simulink model "AFASClosedloopSim"  (R2023a)
settings: Solver=FixedStepAuto  StartTime=0.0  StopTime=600  FixedStep=1/240  RelTol=1e-5
PreLoadFcn:
  | [aircraft, state] = astDehavillandBeaver();
  | thrustX = getCoefficient(aircraft,"CX","Propeller",Component="Propeller");
InitFcn:
  | AFASClosedloopSimInitialization
model workspace (MATLAB code in the model file + MAT data in the model file):
  AirReferencedVelocity = 1
  AircraftPerformance.time = 0
  AircraftPerformance.signals(1).values = [0 0 -2202]
  AircraftPerformance.signals(1).dimensions = 3
  AircraftPerformance.signals(1).label = 'CSTATE'
  AircraftPerformance.signals(1).blockName = 'asb6DOFAirframeTemplate/6DOF EOM/6DOF (Euler Angles)/xe,ye,ze'
  AircraftPerformance.signals(1).stateName = ''
  AircraftPerformance.signals(1).inReferencedModel = 0
  AircraftPerformance.signals(1).sampleTime = [0 0]
  AircraftPerformance.signals(2).values = [0.128665353089 0.259337659946 -0.178947917154]
  AircraftPerformance.signals(2).dimensions = 3
  AircraftPerformance.signals(2).label = 'CSTATE'
  AircraftPerformance.signals(2).blockName = 'asb6DOFAirframeTemplate/6DOF EOM/6DOF (Euler Angles)/Calculate DCM &
    | Euler Angles/phi
    | theta
    | psi'
  AircraftPerformance.signals(2).stateName = ''
  AircraftPerformance.signals(2).inReferencedModel = 0
  AircraftPerformance.signals(2).sampleTime = [0 0]
  AircraftPerformance.signals(3).values = [36.9119692666 8.10720863264 8.82591882596]
  AircraftPerformance.signals(3).dimensions = 3
  AircraftPerformance.signals(3).label = 'CSTATE'
  AircraftPerformance.signals(3).blockName = 'asb6DOFAirframeTemplate/6DOF EOM/6DOF (Euler Angles)/ub,vb,wb'
  AircraftPerformance.signals(3).stateName = ''
  AircraftPerformance.signals(3).inReferencedModel = 0
  AircraftPerformance.signals(3).sampleTime = [0 0]
  AircraftPerformance.signals(4).values = [0 0 0]
  AircraftPerformance.signals(4).dimensions = 3
  AircraftPerformance.signals(4).label = 'CSTATE'
  AircraftPerformance.signals(4).blockName = 'asb6DOFAirframeTemplate/6DOF EOM/6DOF (Euler Angles)/p,q,r '
  AircraftPerformance.signals(4).stateName = ''
  AircraftPerformance.signals(4).inReferencedModel = 0
  AircraftPerformance.signals(4).sampleTime = [0 0]
  AircraftPerformance.signals(5).values = [0 0]
  AircraftPerformance.signals(5).dimensions = 2
  AircraftPerformance.signals(5).label = 'CSTATE'
  AircraftPerformance.signals(5).blockName = 'asb6DOFAirframeTemplate/Environment Model/Dryden Wind Turbulence Model 
    | (Continuous (+q +r))/Filters on velocities/Hwgw(s)/wg_p1'
  AircraftPerformance.signals(5).stateName = ''
  AircraftPerformance.signals(5).inReferencedModel = 0
  AircraftPerformance.signals(5).sampleTime = [0 0]
  AircraftPerformance.signals(6).values = [0 0]
  AircraftPerformance.signals(6).dimensions = 2
  AircraftPerformance.signals(6).label = 'CSTATE'
  AircraftPerformance.signals(6).blockName = 'asb6DOFAirframeTemplate/Environment Model/Dryden Wind Turbulence Model 
    | (Continuous (+q +r))/Filters on velocities/Hwgw(s)/wg_p2'
  AircraftPerformance.signals(6).stateName = ''
  AircraftPerformance.signals(6).inReferencedModel = 0
  AircraftPerformance.signals(6).sampleTime = [0 0]
  AircraftPerformance.signals(7).values = [0 0]
  AircraftPerformance.signals(7).dimensions = 2
  AircraftPerformance.signals(7).label = 'CSTATE'
  AircraftPerformance.signals(7).blockName = 'asb6DOFAirframeTemplate/Environment Model/Dryden Wind Turbulence Model 
    | (Continuous (+q +r))/Filters on velocities/Hvgw(s)/vg_p1'
  AircraftPerformance.signals(7).stateName = ''
  AircraftPerformance.signals(7).inReferencedModel = 0
  AircraftPerformance.signals(7).sampleTime = [0 0]
  AircraftPerformance.signals(8).values = [0 0]
  AircraftPerformance.signals(8).dimensions = 2
  AircraftPerformance.signals(8).label = 'CSTATE'
  AircraftPerformance.signals(8).blockName = 'asb6DOFAirframeTemplate/Environment Model/Dryden Wind Turbulence Model 
    | (Continuous (+q +r))/Filters on velocities/Hvgw(s)/vgw_p2'
  AircraftPerformance.signals(8).stateName = ''
  AircraftPerformance.signals(8).inReferencedModel = 0
  AircraftPerformance.signals(8).sampleTime = [0 0]
  AircraftPerformance.signals(9).values = [0 0]
  AircraftPerformance.signals(9).dimensions = 2
  AircraftPerformance.signals(9).label = 'CSTATE'
  AircraftPerformance.signals(9).blockName = 'asb6DOFAirframeTemplate/Environment Model/Dryden Wind Turbulence Model 
    | (Continuous (+q +r))/Filters on velocities/Hugw(s)/ug_p'
  AircraftPerformance.signals(9).stateName = ''
  AircraftPerformance.signals(9).inReferencedModel = 0
  AircraftPerformance.signals(9).sampleTime = [0 0]
  AircraftPerformance.signals(10).values = [0 0]
  AircraftPerformance.signals(10).dimensions = 2
  AircraftPerformance.signals(10).label = 'CSTATE'
  AircraftPerformance.signals(10).blockName = 'asb6DOFAirframeTemplate/Environment Model/Dryden Wind Turbulence Model 
    | (Continuous (+q +r))/Filters on angular rates/Hrgw/rgw_p'
  AircraftPerformance.signals(10).stateName = ''
  AircraftPerformance.signals(10).inReferencedModel = 0
  AircraftPerformance.signals(10).sampleTime = [0 0]
  AircraftPerformance.signals(11).values = [0 0]
  AircraftPerformance.signals(11).dimensions = 2
  AircraftPerformance.signals(11).label = 'CSTATE'
  AircraftPerformance.signals(11).blockName = 'asb6DOFAirframeTemplate/Environment Model/Dryden Wind Turbulence Model 
    | (Continuous (+q +r))/Filters on angular rates/Hqgw/qgw_p'
  AircraftPerformance.signals(11).stateName = ''
  AircraftPerformance.signals(11).inReferencedModel = 0
  AircraftPerformance.signals(11).sampleTime = [0 0]
  AircraftPerformance.signals(12).values = [0 0]
  AircraftPerformance.signals(12).dimensions = 2
  AircraftPerformance.signals(12).label = 'CSTATE'
  AircraftPerformance.signals(12).blockName = 'asb6DOFAirframeTemplate/Environment Model/Dryden Wind Turbulence Model 
    | (Continuous (+q +r))/Filters on angular rates/Hpgw/pgw_p'
  AircraftPerformance.signals(12).stateName = ''
  AircraftPerformance.signals(12).inReferencedModel = 0
  AircraftPerformance.signals(12).sampleTime = [0 0]
  AircraftPerformance.unnamed = 0
  AircraftPerformance.type = 0
  CurrentWaypoint = 1
  FCCLatDirMode = 1
  FCCVerticalMode = 1
  FlightPlan = 1
  LookaheadDis = 15
  NextWaypoint = 1
  NumofWaypoint = 1
  OwnshipAircraftID = 1
  PreWaypoint = 1
  PreviousWaypoint = Simulink.Parameter
  PreviousWaypoint.DataType = 'auto'
  PreviousWaypoint.Complexity = 'real'
  PreviousWaypoint.Dimensions = [0 0]
  TrajectoryChange = 1
  WaypointType = 1
  inputs0.time = 0
  inputs0.signals(1).dimensions = 1
  inputs0.signals(1).values = -0.104711430294
  inputs0.signals(2).dimensions = 1
  inputs0.signals(2).values = -0.0698725229544
  inputs0.signals(3).dimensions = 1
  inputs0.signals(3).values = -0.000215042330254
  states.time = 0
  states.signals(1).values = 0
  states.signals(1).dimensions = 1
  states.signals(1).label = 'CSTATE'
  states.signals(1).blockName = 'asb6DOFAirframeTemplate/6DOF EOM/6DOF (Euler Angles)/xe,ye,ze'
  states.signals(1).stateName = 'Xe'
  states.signals(1).inReferencedModel = 0
  states.signals(1).sampleTime = [0 0]
  states.signals(2).values = 0
  states.signals(2).dimensions = 1
  states.signals(2).label = 'CSTATE'
  states.signals(2).blockName = 'asb6DOFAirframeTemplate/6DOF EOM/6DOF (Euler Angles)/xe,ye,ze'
  states.signals(2).stateName = 'Ye'
  states.signals(2).inReferencedModel = 0
  states.signals(2).sampleTime = [0 0]
  states.signals(3).values = -2202
  states.signals(3).dimensions = 1
  states.signals(3).label = 'CSTATE'
  states.signals(3).blockName = 'asb6DOFAirframeTemplate/6DOF EOM/6DOF (Euler Angles)/xe,ye,ze'
  states.signals(3).stateName = 'Ze'
  states.signals(3).inReferencedModel = 0
  states.signals(3).sampleTime = [0 0]
  states.signals(4).values = 0.128665353089
  states.signals(4).dimensions = 1
  states.signals(4).label = 'CSTATE'
  states.signals(4).blockName = 'asb6DOFAirframeTemplate/6DOF EOM/6DOF (Euler Angles)/Calculate DCM &
    | Euler Angles/phi
    | theta
    | psi'
  states.signals(4).stateName = 'phi'
  states.signals(4).inReferencedModel = 0
  states.signals(4).sampleTime = [0 0]
  states.signals(5).values = 0.259337659946
  states.signals(5).dimensions = 1
  states.signals(5).label = 'CSTATE'
  states.signals(5).blockName = 'asb6DOFAirframeTemplate/6DOF EOM/6DOF (Euler Angles)/Calculate DCM &
    | Euler Angles/phi
    | theta
    | psi'
  states.signals(5).stateName = 'theta'
  states.signals(5).inReferencedModel = 0
  states.signals(5).sampleTime = [0 0]
  states.signals(6).values = -0.178947917154
  states.signals(6).dimensions = 1
  states.signals(6).label = 'CSTATE'
  states.signals(6).blockName = 'asb6DOFAirframeTemplate/6DOF EOM/6DOF (Euler Angles)/Calculate DCM &
    | Euler Angles/phi
    | theta
    | psi'
  states.signals(6).stateName = 'psi'
  states.signals(6).inReferencedModel = 0
  states.signals(6).sampleTime = [0 0]
  states.signals(7).values = 36.9119692666
  states.signals(7).dimensions = 1
  states.signals(7).label = 'CSTATE'
  states.signals(7).blockName = 'asb6DOFAirframeTemplate/6DOF EOM/6DOF (Euler Angles)/ub,vb,wb'
  states.signals(7).stateName = 'Ubody'
  states.signals(7).inReferencedModel = 0
  states.signals(7).sampleTime = [0 0]
  states.signals(8).values = 8.10720863264
  states.signals(8).dimensions = 1
  states.signals(8).label = 'CSTATE'
  states.signals(8).blockName = 'asb6DOFAirframeTemplate/6DOF EOM/6DOF (Euler Angles)/ub,vb,wb'
  states.signals(8).stateName = 'Vbody'
  states.signals(8).inReferencedModel = 0
  states.signals(8).sampleTime = [0 0]
  states.signals(9).values = 8.82591882596
  states.signals(9).dimensions = 1
  states.signals(9).label = 'CSTATE'
  states.signals(9).blockName = 'asb6DOFAirframeTemplate/6DOF EOM/6DOF (Euler Angles)/ub,vb,wb'
  states.signals(9).stateName = 'Wbody'
  states.signals(9).inReferencedModel = 0
  states.signals(9).sampleTime = [0 0]
  states.signals(10).values = 0
  states.signals(10).dimensions = 1
  states.signals(10).label = 'CSTATE'
  states.signals(10).blockName = 'asb6DOFAirframeTemplate/6DOF EOM/6DOF (Euler Angles)/p,q,r '
  states.signals(10).stateName = 'p'
  states.signals(10).inReferencedModel = 0
  states.signals(10).sampleTime = [0 0]
  states.signals(11).values = 0
  states.signals(11).dimensions = 1
  states.signals(11).label = 'CSTATE'
  states.signals(11).blockName = 'asb6DOFAirframeTemplate/6DOF EOM/6DOF (Euler Angles)/p,q,r '
  states.signals(11).stateName = 'q'
  states.signals(11).inReferencedModel = 0
  states.signals(11).sampleTime = [0 0]
  states.signals(12).values = 0
  states.signals(12).dimensions = 1
  states.signals(12).label = 'CSTATE'
  states.signals(12).blockName = 'asb6DOFAirframeTemplate/6DOF EOM/6DOF (Euler Angles)/p,q,r '
  states.signals(12).stateName = 'r'
  states.signals(12).inReferencedModel = 0
  states.signals(12).sampleTime = [0 0]
  states.signals(13).values = [0 0]
  states.signals(13).dimensions = 2
  states.signals(13).label = 'CSTATE'
  states.signals(13).blockName = 'asb6DOFAirframeTemplate/Environment Model/Dryden Wind Turbulence Model 
    | (Continuous (+q +r))/Filters on velocities/Hwgw(s)/wg_p1'
  states.signals(13).stateName = ''
  states.signals(13).inReferencedModel = 0
  states.signals(13).sampleTime = [0 0]
  states.signals(14).values = [0 0]
  states.signals(14).dimensions = 2
  states.signals(14).label = 'CSTATE'
  states.signals(14).blockName = 'asb6DOFAirframeTemplate/Environment Model/Dryden Wind Turbulence Model 
    | (Continuous (+q +r))/Filters on velocities/Hwgw(s)/wg_p2'
  states.signals(14).stateName = ''
  states.signals(14).inReferencedModel = 0
  states.signals(14).sampleTime = [0 0]
  states.signals(15).values = [0 0]
  states.signals(15).dimensions = 2
  states.signals(15).label = 'CSTATE'
  states.signals(15).blockName = 'asb6DOFAirframeTemplate/Environment Model/Dryden Wind Turbulence Model 
    | (Continuous (+q +r))/Filters on velocities/Hvgw(s)/vg_p1'
  states.signals(15).stateName = ''
  states.signals(15).inReferencedModel = 0
  states.signals(15).sampleTime = [0 0]
  states.signals(16).values = [0 0]
  states.signals(16).dimensions = 2
  states.signals(16).label = 'CSTATE'
  states.signals(16).blockName = 'asb6DOFAirframeTemplate/Environment Model/Dryden Wind Turbulence Model 
    | (Continuous (+q +r))/Filters on velocities/Hvgw(s)/vgw_p2'
  states.signals(16).stateName = ''
  states.signals(16).inReferencedModel = 0
  states.signals(16).sampleTime = [0 0]
  states.signals(17).values = [0 0]
  states.signals(17).dimensions = 2
  states.signals(17).label = 'CSTATE'
  states.signals(17).blockName = 'asb6DOFAirframeTemplate/Environment Model/Dryden Wind Turbulence Model 
    | (Continuous (+q +r))/Filters on velocities/Hugw(s)/ug_p'
  states.signals(17).stateName = ''
  states.signals(17).inReferencedModel = 0
  states.signals(17).sampleTime = [0 0]
  states.signals(18).values = [0 0]
  states.signals(18).dimensions = 2
  states.signals(18).label = 'CSTATE'
  states.signals(18).blockName = 'asb6DOFAirframeTemplate/Environment Model/Dryden Wind Turbulence Model 
    | (Continuous (+q +r))/Filters on angular rates/Hrgw/rgw_p'
  states.signals(18).stateName = ''
  states.signals(18).inReferencedModel = 0
  states.signals(18).sampleTime = [0 0]
  states.signals(19).values = [0 0]
  states.signals(19).dimensions = 2
  states.signals(19).label = 'CSTATE'
  states.signals(19).blockName = 'asb6DOFAirframeTemplate/Environment Model/Dryden Wind Turbulence Model 
    | (Continuous (+q +r))/Filters on angular rates/Hqgw/qgw_p'
  states.signals(19).stateName = ''
  states.signals(19).inReferencedModel = 0
  states.signals(19).sampleTime = [0 0]
  states.signals(20).values = [0 0]
  states.signals(20).dimensions = 2
  states.signals(20).label = 'CSTATE'
  states.signals(20).blockName = 'asb6DOFAirframeTemplate/Environment Model/Dryden Wind Turbulence Model 
    | (Continuous (+q +r))/Filters on angular rates/Hpgw/pgw_p'
  states.signals(20).stateName = ''
  states.signals(20).inReferencedModel = 0
  states.signals(20).sampleTime = [0 0]
  states0.time = 0
  states0.signals(1).values = [0 0 -2202]
  states0.signals(1).dimensions = 3
  states0.signals(1).label = 'CSTATE'
  states0.signals(1).blockName = 'asb6DOFAirframeTemplate/6DOF EOM/6DOF (Euler Angles)/xe,ye,ze'
  states0.signals(1).stateName = ''
  states0.signals(1).inReferencedModel = 0
  states0.signals(1).sampleTime = [0 0]
  states0.signals(2).values = [0.128665353089 0.259337659946 -0.178947917154]
  states0.signals(2).dimensions = 3
  states0.signals(2).label = 'CSTATE'
  states0.signals(2).blockName = 'asb6DOFAirframeTemplate/6DOF EOM/6DOF (Euler Angles)/Calculate DCM &
    | Euler Angles/phi
    | theta
    | psi'
  states0.signals(2).stateName = ''
  states0.signals(2).inReferencedModel = 0
  states0.signals(2).sampleTime = [0 0]
  states0.signals(3).values = [36.9119692666 8.10720863264 8.82591882596]
  states0.signals(3).dimensions = 3
  states0.signals(3).label = 'CSTATE'
  states0.signals(3).blockName = 'asb6DOFAirframeTemplate/6DOF EOM/6DOF (Euler Angles)/ub,vb,wb'
  states0.signals(3).stateName = ''
  states0.signals(3).inReferencedModel = 0
  states0.signals(3).sampleTime = [0 0]
  states0.signals(4).values = [0 0 0]
  states0.signals(4).dimensions = 3
  states0.signals(4).label = 'CSTATE'
  states0.signals(4).blockName = 'asb6DOFAirframeTemplate/6DOF EOM/6DOF (Euler Angles)/p,q,r '
  states0.signals(4).stateName = ''
  states0.signals(4).inReferencedModel = 0
  states0.signals(4).sampleTime = [0 0]
  states0.signals(5).values = [0 0]
  states0.signals(5).dimensions = 2
  states0.signals(5).label = 'CSTATE'
  states0.signals(5).blockName = 'asb6DOFAirframeTemplate/Environment Model/Dryden Wind Turbulence Model 
    | (Continuous (+q +r))/Filters on velocities/Hwgw(s)/wg_p1'
  states0.signals(5).stateName = ''
  states0.signals(5).inReferencedModel = 0
  states0.signals(5).sampleTime = [0 0]
  states0.signals(6).values = [0 0]
  states0.signals(6).dimensions = 2
  states0.signals(6).label = 'CSTATE'
  states0.signals(6).blockName = 'asb6DOFAirframeTemplate/Environment Model/Dryden Wind Turbulence Model 
    | (Continuous (+q +r))/Filters on velocities/Hwgw(s)/wg_p2'
  states0.signals(6).stateName = ''
  states0.signals(6).inReferencedModel = 0
  states0.signals(6).sampleTime = [0 0]
  states0.signals(7).values = [0 0]
  states0.signals(7).dimensions = 2
  states0.signals(7).label = 'CSTATE'
  states0.signals(7).blockName = 'asb6DOFAirframeTemplate/Environment Model/Dryden Wind Turbulence Model 
    | (Continuous (+q +r))/Filters on velocities/Hvgw(s)/vg_p1'
  states0.signals(7).stateName = ''
  states0.signals(7).inReferencedModel = 0
  states0.signals(7).sampleTime = [0 0]
  states0.signals(8).values = [0 0]
  states0.signals(8).dimensions = 2
  states0.signals(8).label = 'CSTATE'
  states0.signals(8).blockName = 'asb6DOFAirframeTemplate/Environment Model/Dryden Wind Turbulence Model 
    | (Continuous (+q +r))/Filters on velocities/Hvgw(s)/vgw_p2'
  states0.signals(8).stateName = ''
  states0.signals(8).inReferencedModel = 0
  states0.signals(8).sampleTime = [0 0]
  states0.signals(9).values = [0 0]
  states0.signals(9).dimensions = 2
  states0.signals(9).label = 'CSTATE'
  states0.signals(9).blockName = 'asb6DOFAirframeTemplate/Environment Model/Dryden Wind Turbulence Model 
    | (Continuous (+q +r))/Filters on velocities/Hugw(s)/ug_p'
  states0.signals(9).stateName = ''
  states0.signals(9).inReferencedModel = 0
  states0.signals(9).sampleTime = [0 0]
  states0.signals(10).values = [0 0]
  states0.signals(10).dimensions = 2
  states0.signals(10).label = 'CSTATE'
  states0.signals(10).blockName = 'asb6DOFAirframeTemplate/Environment Model/Dryden Wind Turbulence Model 
    | (Continuous (+q +r))/Filters on angular rates/Hrgw/rgw_p'
  states0.signals(10).stateName = ''
  states0.signals(10).inReferencedModel = 0
  states0.signals(10).sampleTime = [0 0]
  states0.signals(11).values = [0 0]
  states0.signals(11).dimensions = 2
  states0.signals(11).label = 'CSTATE'
  states0.signals(11).blockName = 'asb6DOFAirframeTemplate/Environment Model/Dryden Wind Turbulence Model 
    | (Continuous (+q +r))/Filters on angular rates/Hqgw/qgw_p'
  states0.signals(11).stateName = ''
  states0.signals(11).inReferencedModel = 0
  states0.signals(11).sampleTime = [0 0]
  states0.signals(12).values = [0 0]
  states0.signals(12).dimensions = 2
  states0.signals(12).label = 'CSTATE'
  states0.signals(12).blockName = 'asb6DOFAirframeTemplate/Environment Model/Dryden Wind Turbulence Model 
    | (Continuous (+q +r))/Filters on angular rates/Hpgw/pgw_p'
  states0.signals(12).stateName = ''
  states0.signals(12).inReferencedModel = 0
  states0.signals(12).sampleTime = [0 0]
  other statements: initialize6DOFSkyHogg;
values from neighbouring files (symbols this model uses):
  alt_ft = 1000    [AFASClosedloopSimInitialization.m]
  alt_hold_av = 1.5    [AFASClosedloopSimInitialization.m]
  alt_hold_hold = 0.1    [AFASClosedloopSimInitialization.m]
  alt_hold_vs = 0.58    [AFASClosedloopSimInitialization.m]
  alt_m = 304.8    [AFASClosedloopSimInitialization.m]
  AT_lead_T1 = 1    [AFASClosedloopSimInitialization.m]
  AT_lead_T2 = 1    [AFASClosedloopSimInitialization.m]
  AT_spd_hold_cmpst = 0.5    [AFASClosedloopSimInitialization.m]
  AT_spd_hold_ptch_tau_gain = 0.15    [AFASClosedloopSimInitialization.m]
  AT_spd_hold_rate_damping_gain = 10    [AFASClosedloopSimInitialization.m]
  AT_spd_hold_tas_lp_tau = 5.0    (= 5)    [AFASClosedloopSimInitialization.m]
  AT_spd_hold_tas_val_lp_tau = 0.5    [AFASClosedloopSimInitialization.m]
  AT_struct_den = 1    [AFASClosedloopSimInitialization.m]
  AT_struct_num = 1    [AFASClosedloopSimInitialization.m]
  AT_svo_composite = 1    [AFASClosedloopSimInitialization.m]
  av_hp_fltr_tau = 10    [AFASClosedloopSimInitialization.m]
  av_lp_fltr_tau = 0.5    [AFASClosedloopSimInitialization.m]
  cas_mps = 72.0222    [AFASClosedloopSimInitialization.m]
  Cl0 = 5.910000000000000e-04    (= 0.000591)    [AFASClosedloopSimInitialization.m]
  Cl_beta = -0.0618    [AFASClosedloopSimInitialization.m]
  Cl_da = -0.0992    [AFASClosedloopSimInitialization.m]
  Cl_da_alpha = -0.0827    [AFASClosedloopSimInitialization.m]
  Cl_dr = 0.0069    [AFASClosedloopSimInitialization.m]
  Cl_p = -0.5045    [AFASClosedloopSimInitialization.m]
  Cl_r = 0.1695    [AFASClosedloopSimInitialization.m]
  Cm0 = 0.0945    [AFASClosedloopSimInitialization.m]
  Cm_alpha = -0.6028    [AFASClosedloopSimInitialization.m]
  Cm_alpha2 = -2.1400    (= -2.14)    [AFASClosedloopSimInitialization.m]
  Cm_beta2 = 0.6921    [AFASClosedloopSimInitialization.m]
  Cm_de = -1.9210    (= -1.921)    [AFASClosedloopSimInitialization.m]
  Cm_df = 0.4072    [AFASClosedloopSimInitialization.m]
  Cm_q = -15.5600    (= -15.56)    [AFASClosedloopSimInitialization.m]
  Cm_r = -0.3118    [AFASClosedloopSimInitialization.m]
  Cn0 = -0.0031    [AFASClosedloopSimInitialization.m]
  Cn_beta = 0.0067    [AFASClosedloopSimInitialization.m]
  Cn_beta3 = 0.1373    [AFASClosedloopSimInitialization.m]
  Cn_da = -0.0039    [AFASClosedloopSimInitialization.m]
  Cn_dr = -0.0827    [AFASClosedloopSimInitialization.m]
  Cn_p = -0.1585    [AFASClosedloopSimInitialization.m]
  Cn_q = 0.1595    [AFASClosedloopSimInitialization.m]
  Cn_r = -0.1112    [AFASClosedloopSimInitialization.m]
  Cx0 = -0.0355    [AFASClosedloopSimInitialization.m]
  Cx_alpha = 0.0029    [AFASClosedloopSimInitialization.m]
  Cx_alpha2 = 5.4590    (= 5.459)    [AFASClosedloopSimInitialization.m]
  Cx_alpha3 = -5.1620    (= -5.162)    [AFASClosedloopSimInitialization.m]
  Cx_df = -0.0945    [AFASClosedloopSimInitialization.m]
  Cx_df_alpha = 1.1060    (= 1.106)    [AFASClosedloopSimInitialization.m]
  Cx_dr = 0.0341    [AFASClosedloopSimInitialization.m]
  Cx_q = -0.6748    [AFASClosedloopSimInitialization.m]
  Cy0 = -0.0022    [AFASClosedloopSimInitialization.m]
  Cy_beta = -0.7678    [AFASClosedloopSimInitialization.m]
  Cy_da = -0.0296    [AFASClosedloopSimInitialization.m]
  Cy_dr = 0.1158    [AFASClosedloopSimInitialization.m]
  Cy_dr_alpha = 0.5238    [AFASClosedloopSimInitialization.m]
  Cy_p = -0.1240    (= -0.124)    [AFASClosedloopSimInitialization.m]
  Cy_r = 0.3666    [AFASClosedloopSimInitialization.m]
  Cz0 = -0.0550    (= -0.055)    [AFASClosedloopSimInitialization.m]
  Cz_alpha = -5.5780    (= -5.578)    [AFASClosedloopSimInitialization.m]
  Cz_alpha3 = 3.4420    (= 3.442)    [AFASClosedloopSimInitialization.m]
  Cz_de = -0.3980    (= -0.398)    [AFASClosedloopSimInitialization.m]
  Cz_de_beta = -15.9300    (= -15.93)    [AFASClosedloopSimInitialization.m]
  Cz_df = -1.3770    (= -1.377)    [AFASClosedloopSimInitialization.m]
  Cz_df_alpha = -1.2610    (= -1.261)    [AFASClosedloopSimInitialization.m]
  Cz_q = -2.9880    (= -2.988)    [AFASClosedloopSimInitialization.m]
  hdg_select_hdg_rate_capt = 0.2    [AFASClosedloopSimInitialization.m]
  hdg_select_hdg_rate_damping = 1    [AFASClosedloopSimInitialization.m]
  hdg_select_hdg_rate_track = 0.05    [AFASClosedloopSimInitialization.m]
  lat_accel_aug_lp_tau = 10    [AFASClosedloopSimInitialization.m]
  ltrl_acc_gain = -0.04    [AFASClosedloopSimInitialization.m]
  ltrl_acc_lp_tau = 0.5    [AFASClosedloopSimInitialization.m]
  mach = 0.213    [AFASClosedloopSimInitialization.m]
  OwnshipAircraftConfig = 0    [AFASClosedloopSimInitialization.m]
  pitch_att_gain = 0.7    [AFASClosedloopSimInitialization.m]
  pitch_lead_T1 = 1    [AFASClosedloopSimInitialization.m]
  pitch_lead_T2 = 1    [AFASClosedloopSimInitialization.m]
  pitch_rate_gain = -1400    [AFASClosedloopSimInitialization.m]
  pitch_rate_gain_GAIN1 = -56    [AFASClosedloopSimInitialization.m]
  pitch_rate_gain_GAIN2 = -52.25    [AFASClosedloopSimInitialization.m]
  pitch_rate_gain_IAS1 = 100    [AFASClosedloopSimInitialization.m]
  pitch_rate_gain_IAS2 = 380    [AFASClosedloopSimInitialization.m]
  pitch_rate_gain_schd = [4.24        2.80        2.24        1.68        1.44        1.22        0.97        0.85        0.77        0.72        0.66    ] * 1000    [AFASClosedloopSimInitialization.m]
  pitch_rate_gain_spd = [85          100.0       120.00      140.00      160.00      180.00      200.00      220.00      240.00      260.00      275.00  ] * 0.5144444    [AFASClosedloopSimInitialization.m]
  pitch_schedule_type = 3    [AFASClosedloopSimInitialization.m]
  pitch_struct_den = 1    [AFASClosedloopSimInitialization.m]
  pitch_struct_num = 1    [AFASClosedloopSimInitialization.m]
  pitch_svo_composite = 1    [AFASClosedloopSimInitialization.m]
  pitch_svo_integral = 0.6    [AFASClosedloopSimInitialization.m]
  roll_att_gain = 0.45    [AFASClosedloopSimInitialization.m]
  roll_lead_T1 = 1    [AFASClosedloopSimInitialization.m]
  roll_lead_T2 = 1    [AFASClosedloopSimInitialization.m]
  roll_limit = 30*d2r    (= 0.5235987)    [AFASClosedloopSimInitialization.m]
  roll_rate_gain = 561.5    [AFASClosedloopSimInitialization.m]
  roll_rate_gain_GAIN1 = 57.25    [AFASClosedloopSimInitialization.m]
  roll_rate_gain_GAIN2 = 41.25    [AFASClosedloopSimInitialization.m]
  roll_rate_gain_IAS1 = 100    [AFASClosedloopSimInitialization.m]
  roll_rate_gain_IAS2 = 380    [AFASClosedloopSimInitialization.m]
  roll_rate_gain_schd = [1.30        0.86        0.71        0.63        0.57        0.50        0.46        0.46    ] * 1000    [AFASClosedloopSimInitialization.m]
  roll_rate_gain_spd = [85.00       100.00      120.00      140.00      160.00      200.00      220.00      275.00  ] * 0.5144444    [AFASClosedloopSimInitialization.m]
  roll_schedule_type = 3    [AFASClosedloopSimInitialization.m]
  roll_struct_den = 1    [AFASClosedloopSimInitialization.m]
  roll_struct_num = 1    [AFASClosedloopSimInitialization.m]
  roll_svo_composite = 0.00001    (= 1e-05)    [AFASClosedloopSimInitialization.m]
  roll_svo_integral = 0.6    [AFASClosedloopSimInitialization.m]
  tas_mps = 73.051    [AFASClosedloopSimInitialization.m]
  TGR = 0.25    [AFASClosedloopSimInitialization.m]
  wingrock_enable_alt = 20000    [AFASClosedloopSimInitialization.m]
  wingrock_enable_mach = 0.6    [AFASClosedloopSimInitialization.m]
  wingrock_lookup_data = [2 2  1 1]    [AFASClosedloopSimInitialization.m]
  wingrock_lookup_row = [0 2 5 10]*pi/180    [AFASClosedloopSimInitialization.m]
  wingrock_schedule_type = 3    [AFASClosedloopSimInitialization.m]
  yaw_rate_gain = 15521    [AFASClosedloopSimInitialization.m]
  yaw_rate_gain_GAIN1 = 37.8352    [AFASClosedloopSimInitialization.m]
  yaw_rate_gain_GAIN2 = 24.2654    [AFASClosedloopSimInitialization.m]
  yaw_rate_gain_IAS1 = 100    [AFASClosedloopSimInitialization.m]
  yaw_rate_gain_IAS2 = 340    [AFASClosedloopSimInitialization.m]
  yaw_rate_gain_piecewise_schd = [7.68	5.98		3.22	2.59		1.78 ... (first row only)    [AFASClosedloopSimInitialization.m]
  yaw_rate_gain_schd = [15521    11532   11532   10115   8951.7  7831.7  6829.2  5739.3  4506.7  3317.9  3391.5  2103.9  1404.5  994.3226]    [AFASClosedloopSimInitialization.m]
  yaw_rate_gain_spd = [90       97      106     111     118     127     136     149     165     187     192     228     264     295     ] * 0.5144444    [AFASClosedloopSimInitialization.m]
  yaw_rate_hp_tau = 1.8    [AFASClosedloopSimInitialization.m]
  yd_lead_T1 = yd_a * yd_lead_T2    [AFASClosedloopSimInitialization.m]
  ... (+7 more)
undefined symbols (not defined in the file or in its folder): aircraft, DiscIntNeverNeededParam, Earth, F, Light, MIL, sigbuilder_block, state, WGS84
libraries: aerolibasang x4, aerolibactuator x4, aerolibguid x2, simulink x2, dspnetwork x2, etargetslib x2, shared6dof x1, aerolibadyn x1, aerolibatmos2 x1, aerolibwind2 x1, aerolibtransform2 x1, sharedtransform x1
(part 1 of 4)
settings Model: Creator=Albatrossai  LastModifiedBy=Albatrossai
settings SolverCC: AlgebraicLoopSolver=TrustRegion  AutoInsertRateTranBlk=on  InsertRTBMode=Never (minimum delay)  MinimalZcImpactIntegration=on  MaxZcPerStep=1
settings DataIOCC: ExternalInput=inputs0  InitialState=states  SaveFormat=Array  SaveOutput=off
settings OptimizationCC: OptimizeBlockIOStorage=off  EnhancedBackFolding=on  StrengthReduction=on  InitFltsAndDblsToZero=on  OptimizeDataStoreBuffers=off  BusAssignmentInplaceUpdate=off
settings DebuggingCC: WriteAfterWriteMsg=DisableAll  AlgebraicLoopMsg=none  FcnCallInpInsideContextMsg=warning  UniqueDataStoreMsg=error  RootOutportRequireBusObject=none  StateNameClashWarn=warning  StrictBusMsg=ErrorOnBusTreatedAsVector  SFUnexpectedBacktrackingDiag=warning  SFNoUnconditionalDefaultTransitionDiag=warning  SFExecutionAtInitializationDiag=none  ArithmeticOperatorsInVariantConditions=warning
settings ModelReferenceCC: EnableRefExpFcnMdlSchedulingChecks=on  PropagateSignalLabelsOutOfModel=off
settings SFSimCC: SimCustomHeaderCode="#include \"AFAS_func.h\""  SimUserSources=AFAS_func.c  SimUseLocalCustomCode=off
settings RTWCC: Description=Create Visual C/C++ Solution File for Simulink Coder  GenCodeOnly=on  TemplateMakefile=RTW.MSVCBuild  GenerateReport=on  RTWUseLocalCustomCode=off  BuildConfiguration=Debug  LaunchReport=on  DLArmComputeVersion=19.05
settings CodeAppCC: ForceParamTrailComments=on  MATLABSourceComments=on  EnableCustomComments=on

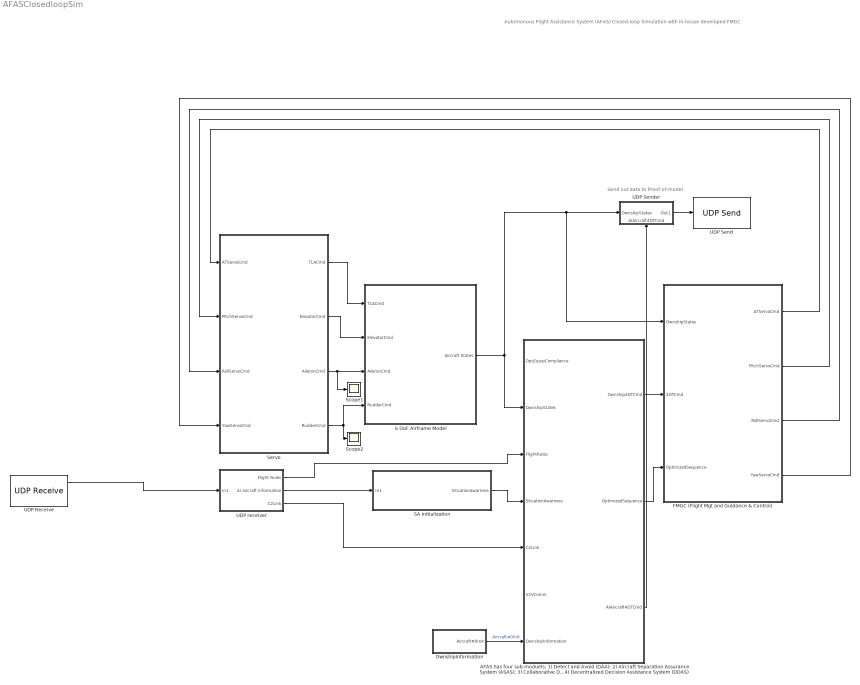
== system AFASClosedloopSim ==
  note: Send out data to Proof-of-model
  note: Automonous Flight Assistance System (AFAS)
      | Closed-loop Simulation with in-house developed FMGC
  6 DoF Airframe Model : Subsystem
  "AFAS has four sub-moduels: 1) Detect and Avoid (DAA); 2) Aircraft Separation Assurance System (ASAS); 3) Collaborative Decision Assistance System (CDAS); 4) Decentralized Decision Assistance System (DDAS) " : Subsystem
  FMGC (Flight Mgt and Guidance & Control) : Subsystem
  OwnshipInformation : Subsystem
  "SA Initialization " : Subsystem
  Scope1 : Scope
  Scope2 : Scope
  Servo : Subsystem
  UDP Receive : dspnetwork/UDP Receive  localURL='0.0.0.0'  localPort=25000  remoteURL='0.0.0.0'  remotePort=-1  recvBufferSize=8192  dims=3  signalDatatype=uint8  isComplex=off  isVarSize=off  showBlockingTime=on  blockingTime=0  sampletime=1/120  blockPlatform=HOST
      settings: LibrarySourceBlock=embeddedtargetslib/Host Communication/UDP Receive
  UDP Send : dspnetwork/UDP Send  remoteURL='255.255.255.255'  remotePort=25000  localURL='0.0.0.0'  localPortSource=Automatically determine  localPort=-1  sendBufferSize=8192  sampletime=-1  blockPlatform=HOST  separateLengthPort=0
      settings: LibrarySourceBlock=embeddedtargetslib/Host Communication/UDP Send
  UDP Sender : Subsystem
      settings: PortSchema="{\"entries\":[{\"content\":{\"sides\":[{\"content\":{\"connectorIds\":[\"In1\"]},\"type\":\"ConnectorPlacement.EquallySpacedRectSide\",\"uuid\":\"0b093b1f-b31a-42a2-93da-f9649bd6b450\"},{\"content\":{\"connectorIds\":[\"Out1\"],\"side\":\"RIGHT\"},\"type\":\"ConnectorPlacement.EquallySpacedRectSide\",\"uuid\":\"1c5e0f47-ef90-489b-9e72-447b6e8b864e\"},{\"content\":{\"side\":\"TOP\"},\"type\":\"ConnectorPlacement.EquallySpacedRectSide\",\"uuid\":\"22e4e857-ae3e-41ac-844b-889b1fa25fe7\"},{\"content\":{\"connectorIds\":[\"In2\"],\"side\":\"BOTTOM\"},\"type\":\"ConnectorPlacement.EquallySpacedRectSide\",\"uuid\":\"a698749d-9d94-4f24-80dc-0c1e62ff27b6\"}]},\"type\":\"ConnectorPlacement.EquallySpacedConnector\",\"uuid\":\"ad223273-0610-4ecf-a702-8df58219ef50\"}],\"packageUris\":[\"http://schema.mathworks.com/mf0/Connector/R2020b\"],\"version\":\"1.0\"}"
  UDP receiver : Subsystem
  wires:
  Servo/4(RudderCmd) -> 6 DoF Airframe Model/4(RudderCmd), Scope2/1
  UDP Sender/1(Out1) -> UDP Send/1
  UDP Receive/1 -> UDP receiver/1(In1)
  6 DoF Airframe Model/1(Aircraft States) -> UDP Sender/1(OwnshipStates), FMGC (Flight Mgt and Guidance & Control)/1(OwnshipStates), "AFAS has four sub-moduels: 1) Detect and Avoid (DAA); 2) Aircraft Separation Assurance System (ASAS); 3) Collaborative Decision Assistance System (CDAS); 4) Decentralized Decision Assistance System (DDAS) "/2(OwnshipStates)
  UDP receiver/2(AI aircraft Information) -> "SA Initialization "/1(In1)
  Servo/1(TLACmd) -> 6 DoF Airframe Model/1(TLACmd)
  UDP receiver/1(Flight Rules) -> "AFAS has four sub-moduels: 1) Detect and Avoid (DAA); 2) Aircraft Separation Assurance System (ASAS); 3) Collaborative Decision Assistance System (CDAS); 4) Decentralized Decision Assistance System (DDAS) "/3(FlightRules)
  Servo/2(ElevatorCmd) -> 6 DoF Airframe Model/2(ElevatorCmd)
  Servo/3(AileronCmd) -> Scope1/1, 6 DoF Airframe Model/3(AileronCmd)
  UDP receiver/3(C2Link) -> "AFAS has four sub-moduels: 1) Detect and Avoid (DAA); 2) Aircraft Separation Assurance System (ASAS); 3) Collaborative Decision Assistance System (CDAS); 4) Decentralized Decision Assistance System (DDAS) "/5(C2Link)
  "SA Initialization "/1(SituationAwarness) -> "AFAS has four sub-moduels: 1) Detect and Avoid (DAA); 2) Aircraft Separation Assurance System (ASAS); 3) Collaborative Decision Assistance System (CDAS); 4) Decentralized Decision Assistance System (DDAS) "/4(SituationAwarness)
  FMGC (Flight Mgt and Guidance & Control)/4(YawServoCmd) -> Servo/4(YawServoCmd)
  "AFAS has four sub-moduels: 1) Detect and Avoid (DAA); 2) Aircraft Separation Assurance System (ASAS); 3) Collaborative Decision Assistance System (CDAS); 4) Decentralized Decision Assistance System (DDAS) "/1(Ownship4DTCmd) -> FMGC (Flight Mgt and Guidance & Control)/2(4DTCmd)
  "AFAS has four sub-moduels: 1) Detect and Avoid (DAA); 2) Aircraft Separation Assurance System (ASAS); 3) Collaborative Decision Assistance System (CDAS); 4) Decentralized Decision Assistance System (DDAS) "/2(OptimizedSequence) -> FMGC (Flight Mgt and Guidance & Control)/3(OptimizedSequence)
  FMGC (Flight Mgt and Guidance & Control)/1(ATServoCmd) -> Servo/1(ATServoCmd)
  FMGC (Flight Mgt and Guidance & Control)/2(PitchServoCmd) -> Servo/2(PitchServoCmd)
  FMGC (Flight Mgt and Guidance & Control)/3(RollServoCmd) -> Servo/3(RollServoCmd)
  "AFAS has four sub-moduels: 1) Detect and Avoid (DAA); 2) Aircraft Separation Assurance System (ASAS); 3) Collaborative Decision Assistance System (CDAS); 4) Decentralized Decision Assistance System (DDAS) "/3(AIAircraft4DTCmd) -> UDP Sender/2(AIAircraft4DTCmd)
  OwnshipInformation/1(Aircraft#0Init) -> "AFAS has four sub-moduels: 1) Detect and Avoid (DAA); 2) Aircraft Separation Assurance System (ASAS); 3) Collaborative Decision Assistance System (CDAS); 4) Decentralized Decision Assistance System (DDAS) "/7(OwnshipInformation)  "Aircraft#0Init"

== system AFASClosedloopSim/6 DoF Airframe Model ==
  note: 6DOF Airframe (De Havilland Beaver)
  note: Environmental Models
  note: Commands
  TLACmd : Inport
  ElevatorCmd : Inport  Port=2
  AileronCmd : Inport  Port=3
  RudderCmd : Inport  Port=4
  6DOF EOM : Subsystem  VariantControl=eom3DOF
  Aerodynamic Model : Subsystem  VariantControl=aeroCONST
  Environment Model : Subsystem  mask(Environment Model){spec=MIL-F-8785C, model=Continuous Dryden (+q -r), W20=5, Wdeg=0, TurbProb=10^-2 - Light, L_high=533.4, Wingspan=4, ts=0.1, Seed=[23341 23342 23343 23344], T_on=off, refAlt=state.GroundHeight}
      mask prompts: spec "aeroblks:aeroblkwind:blockWindTurbulenceModelParamSpecification"; model "aeroblks:aeroblkwind:blockWindTurbulenceModelParamModeltype"; W20 "Wind speed at 6 m defines the low-altitude intensity (m/s):"; Wdeg "Wind direction at 6 m (degrees clockwise from north):"; TurbProb "aeroblks:aeroblkwind:blockWindTurbulenceModelParamProbabilityofexceedanceofhighaltitudeintensity"; L_high "Scale length at medium/high altitudes (m):"; Wingspan "Wingspan (m):"; ts "Band limited noise sample time (sec):"; Seed "aeroblks:aeroblkwind:blockWindTurbulenceModelParamNoiseseedsugvgwgpg"; T_on "aeroblks:aeroblkwind:blockWindTurbulenceModelParamTurbulenceon"; refAlt "Reference height from Earth's surface to Flat Earth frame [m]:"
      mask help: This block contains an athmospheric model, a wind turbulence model, and a gravity model.
      mask Help: helpview(fullfile(docroot,'toolbox','aeroblks','aeroblks.map'), 'environment1');
      mask TypeOptions spec:
      | Dryden Wind Turbulence Model
      | (Continuous (+q +r))/spec
      mask TypeOptions model:
      | Dryden Wind Turbulence Model
      | (Continuous (+q +r))/model
      mask TypeOptions W20:
      | Dryden Wind Turbulence Model
      | (Continuous (+q +r))/W20
      mask TypeOptions Wdeg:
      | Dryden Wind Turbulence Model
      | (Continuous (+q +r))/Wdeg
      mask TypeOptions TurbProb:
      | Dryden Wind Turbulence Model
      | (Continuous (+q +r))/TurbProb
      mask TypeOptions L_high:
      | Dryden Wind Turbulence Model
      | (Continuous (+q +r))/L_high
      mask TypeOptions Wingspan:
      | Dryden Wind Turbulence Model
      | (Continuous (+q +r))/Wingspan
      mask TypeOptions ts:
      | Dryden Wind Turbulence Model
      | (Continuous (+q +r))/ts
      mask TypeOptions Seed:
      | Dryden Wind Turbulence Model
      | (Continuous (+q +r))/Seed
      mask TypeOptions T_on:
      | Dryden Wind Turbulence Model
      | (Continuous (+q +r))/T_on
      mask DialogControl Container4 Prompt: Atmospheric Model
      mask DialogControl Container17 Prompt: 1976 COESA-extended U.S. Standard Atmospheric Model
      mask DialogControl Control6 Prompt: There are no modifiable parameters for COESA.
      mask DialogControl Container6 Prompt: Wind Model
      mask DialogControl Container16 Prompt: Dryden Wind Turbulence Model
      mask DialogControl spec Prompt: Specification:
      mask DialogControl model Prompt: Model type:
      mask DialogControl TurbProb Prompt: Probability of exceedance of high-altitude intensity:
      mask DialogControl Seed Prompt: Noise seeds [ug vg wg pg]:
      mask DialogControl T_on Prompt: Turbulence on
      mask DialogControl Container8 Prompt: Gravity Model
      mask DialogControl Container18 Prompt: World Geodetic System (WGS 84) Gravity Taylor Series Model
      mask Display:
      | image('aeroenvironment.bmp',[.15,.15,.55,.75])
      | port_label('output',1,'Env')
  Mux : Mux  Inputs=3
  Propulsion : Subsystem
      settings: RTWSystemCode=Inline
  Scope : Scope
  Sum1 : Sum  Inputs=|++  InputSameDT=on  SaturateOnIntegerOverflow=on  OutDataTypeStr=Inherit: Same as first input
  Sum2 : Sum  Inputs=|++  InputSameDT=on  SaturateOnIntegerOverflow=on  OutDataTypeStr=Inherit: Same as first input
  Terminator : Terminator
  Throttle : Constant  Value=.5
  Visualization : Subsystem
  Aircraft States : Outport  OutDataTypeStr=double  VectorParamsAs1DForOutWhenUnconnected=off
  wires:
  Mux/1 -> Aerodynamic Model/2(ActuatorCmds)
  Environment Model/1(Env) -> 6DOF EOM/1(Env), Aerodynamic Model/1(Env)
  Sum2/1 -> 6DOF EOM/2(Forces)
  AileronCmd/1 -> Scope/1, Mux/1  "AileronCmd"
  Propulsion/1(F) -> Sum2/2
  6DOF EOM/1(States) -> Environment Model/1(States), Aircraft States/1, Aerodynamic Model/3(States), Visualization/1(States)
  Sum1/1 -> 6DOF EOM/3(Moments)
  Aerodynamic Model/1(F) -> Sum2/1
  Aerodynamic Model/2(M) -> Sum1/1
  Propulsion/2(M) -> Sum1/2
  Throttle/1 -> Propulsion/1(cmd)
  TLACmd/1 -> Terminator/1
  ElevatorCmd/1 -> Mux/2  "ElevatorCmd"
  RudderCmd/1 -> Mux/3  "RudderCmd"

== system AFASClosedloopSim/AFAS has four sub-moduels: 1) Detect and Avoid (DAA); 2) Aircraft Separation Assurance System (ASAS); 3) Collaborative Decision Assistance System (CDAS); 4) Decentralized Decision Assistance System (DDAS)  ==
  OpsEquipCompliance : Inport
  OwnshipStates : Inport  Port=2
  FlightRules : Inport  Port=3
  SituationAwarness : Inport  Port=4
  C2Link : Inport  Port=5
  V2VComm : Inport  Port=6
  OwnshipInformation : Inport  Port=7
  ASAS: Aircraft Separation Assurance System : Subsystem
  CDAS: Collaborative Decision Assistance System : Subsystem
  DAA: Detection and Avoid : Subsystem
  DDAS: Decentralized Decision Assistance System : Subsystem
  Ownship4DTCmd : Outport
  OptimizedSequence : Outport  Port=2
  AIAircraft4DTCmd : Outport  Port=3
  wires:
  C2Link/1 -> DDAS: Decentralized Decision Assistance System/5(C2Link)
  FlightRules/1 -> DDAS: Decentralized Decision Assistance System/1(FlightRules)
  OpsEquipCompliance/1 -> DDAS: Decentralized Decision Assistance System/2(OpsEquipCompliance)
  SituationAwarness/1 -> DDAS: Decentralized Decision Assistance System/3(SituationAwarness)
  OwnshipStates/1 -> DDAS: Decentralized Decision Assistance System/4(OwnshipStates)
  V2VComm/1 -> DDAS: Decentralized Decision Assistance System/6(V2VComm)
  DDAS: Decentralized Decision Assistance System/1(Ownship4DTCmd) -> Ownship4DTCmd/1
  DDAS: Decentralized Decision Assistance System/2(OptimizedSequence) -> OptimizedSequence/1
  DDAS: Decentralized Decision Assistance System/3(AIAircraft4DTCmd) -> AIAircraft4DTCmd/1
  OwnshipInformation/1 -> DDAS: Decentralized Decision Assistance System/7(OwnshipInformation)

== system AFASClosedloopSim/FMGC (Flight Mgt and Guidance & Control) ==
  OwnshipStates : Inport
  4DTCmd : Inport  Port=2
  OptimizedSequence : Inport  Port=3
  AFCC: Albatross.ai Flight Control Computer : Subsystem
  AFMS: Albatross Flight Management System : Subsystem
  Terminator : Terminator
  ATServoCmd : Outport
  PitchServoCmd : Outport  Port=2
  RollServoCmd : Outport  Port=3
  YawServoCmd : Outport  Port=4
  wires:
  OwnshipStates/1 -> AFCC: Albatross.ai Flight Control Computer/3(OwnshipStates), AFMS: Albatross Flight Management System/1(OwnshipStates)
  AFMS: Albatross Flight Management System/2(RMTargets) -> AFCC: Albatross.ai Flight Control Computer/2(RMTargets)
  4DTCmd/1 -> AFMS: Albatross Flight Management System/2(4DTCmd)
  AFCC: Albatross.ai Flight Control Computer/2(PitchServoCmd) -> PitchServoCmd/1
  OptimizedSequence/1 -> Terminator/1
  AFMS: Albatross Flight Management System/1(TMTargets) -> AFCC: Albatross.ai Flight Control Computer/1(TMTargets)
  AFCC: Albatross.ai Flight Control Computer/3(RollServoCmd) -> RollServoCmd/1
  AFCC: Albatross.ai Flight Control Computer/1(ATServoCmd) -> ATServoCmd/1
  AFCC: Albatross.ai Flight Control Computer/4(YawServoCmd) -> YawServoCmd/1

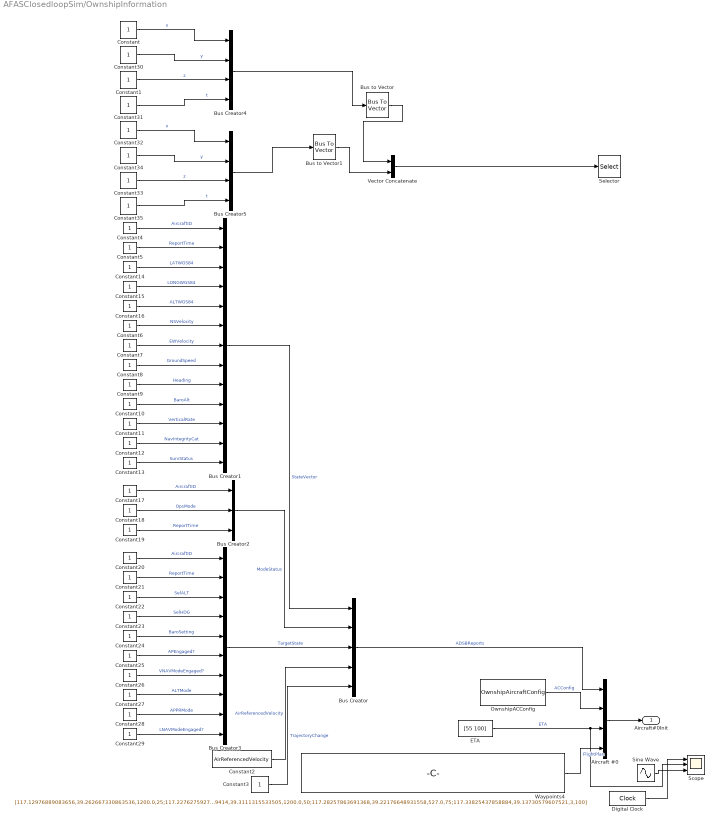
== system AFASClosedloopSim/OwnshipInformation ==
  Aircraft #0 : BusCreator  Inputs=4
  Bus Creator : BusCreator  Inputs=5
  Bus Creator1 : BusCreator  Inputs=13
  Bus Creator2 : BusCreator  Inputs=3
  Bus Creator3 : BusCreator  Inputs=10
  Bus Creator4 : BusCreator  Inputs=4  OutDataTypeStr=Bus: waypoint
  Bus Creator5 : BusCreator  Inputs=4  OutDataTypeStr=Bus: waypoint
  Bus to Vector : BusToVector
  Bus to Vector1 : BusToVector
  Constant{,1,3..35} (35 alike) : Constant
  Constant2 : Constant  Value=AirReferencedVelocity
  Digital Clock : DigitalClock
  ETA : Constant  Value=[55 100]
  OwnshipACConfig : Constant  Value=OwnshipAircraftConfig
  Scope : Scope  NumInputPorts=3
  Selector : Selector  InputPortWidth=8  IndexOptions=Index vector (dialog)  Indices=[1]  OutputSizes=1
  Sine Wave : Sin  SampleTime=0
  Vector Concatenate : Concatenate
  Waypoints4 : Constant  Value=[117.12976889083656,39.262667330863536,1200.0,25;117.22762759279414,39.3111315533505,1200.0,50;117.28257863691368,39.22176648931558,527.0,75;117.33825437858884,39.13730579607521,3,100]
  Aircraft#0Init : Outport
  wires:
  Constant35/1 -> Bus Creator5/4  "t"
  Constant33/1 -> Bus Creator5/3  "z"
  Constant34/1 -> Bus Creator5/2  "y"
  Constant/1 -> Bus Creator4/1  "x"
  Constant30/1 -> Bus Creator4/2  "y"
  Constant1/1 -> Bus Creator4/3  "z"
  Constant31/1 -> Bus Creator4/4  "t"
  Constant32/1 -> Bus Creator5/1  "x"
  Constant3/1 -> Bus Creator/5  "TrajectoryChange"
  Constant4/1 -> Bus Creator1/1  "AircraftID"
  Constant6/1 -> Bus Creator1/6  "NSVelocity"
  Constant5/1 -> Bus Creator1/2  "ReportTime"
  Constant13/1 -> Bus Creator1/13  "SurvStatus"
  Constant14/1 -> Bus Creator1/3  "LATWGS84"
  Constant16/1 -> Bus Creator1/5  "ALTWGS84"
  Constant15/1 -> Bus Creator1/4  "LONGWGS84"
  Constant8/1 -> Bus Creator1/8  "GroundSpeed"
  Constant7/1 -> Bus Creator1/7  "EWVelocity"
  Constant9/1 -> Bus Creator1/9  "Heading"
  ETA/1 -> Scope/2, Aircraft #0/3  "ETA"
  Constant10/1 -> Bus Creator1/10  "BaroAlt"
  Constant12/1 -> Bus Creator1/12  "NavIntegrityCat"
  Constant11/1 -> Bus Creator1/11  "VerticalRate"
  Constant18/1 -> Bus Creator2/2  "OpsMode"
  Constant17/1 -> Bus Creator2/1  "AircraftID"
  Constant2/1 -> Bus Creator/4  "AirReferencedVelocity"
  Constant19/1 -> Bus Creator2/3  "ReportTime"
  Constant21/1 -> Bus Creator3/2  "ReportTime"
  Constant20/1 -> Bus Creator3/1  "AircraftID"
  Constant23/1 -> Bus Creator3/4  "SelHDG"
  Constant22/1 -> Bus Creator3/3  "SelALT"
  Constant25/1 -> Bus Creator3/6  "APEngaged?"
  Constant24/1 -> Bus Creator3/5  "BaroSetting"
  Constant27/1 -> Bus Creator3/8  "ALTMode"
  Constant26/1 -> Bus Creator3/7  "VNAVModeEngaged?"
  Constant29/1 -> Bus Creator3/10  "LNAVModeEngaged?"
  Constant28/1 -> Bus Creator3/9  "APPRMode"
  Vector Concatenate/1 -> Selector/1
  Bus Creator4/1 -> Bus to Vector/1
  Bus Creator5/1 -> Bus to Vector1/1
  Bus Creator1/1 -> Bus Creator/1  "StateVector"
  Bus Creator2/1 -> Bus Creator/2  "ModeStatus"
  Bus Creator3/1 -> Bus Creator/3  "TargetState"
  Bus Creator/1 -> Aircraft #0/1  "ADSBReports"
  OwnshipACConfig/1 -> Aircraft #0/2  "ACConfig"
  Waypoints4/1 -> Aircraft #0/4  "FlightPlan"
  Aircraft #0/1 -> Aircraft#0Init/1
  Bus to Vector/1 -> Vector Concatenate/1
  Bus to Vector1/1 -> Vector Concatenate/2
  Sine Wave/1 -> Scope/3
  Digital Clock/1 -> Scope/1

== system AFASClosedloopSim/SA Initialization  ==
  In1 : Inport
  Bus Creator : BusCreator  Inputs=6
  Bus Selector : BusSelector  OutputSignals=signal1,signal2
  Chart1 : Stateflow chart  TreatAsAtomicUnit=on
  Constant : Constant  Value=0
  Constant1 : Constant
  Subsystem : Subsystem
  Subsystem1 : Subsystem
  Subsystem2 : Subsystem
  Subsystem3 : Subsystem
  Subsystem4 : Subsystem
  Subsystem5 : Subsystem
  Switch : Switch  Criteria=u2 > Threshold  Threshold=1000  SaturateOnIntegerOverflow=off  InputSameDT=off
  Switch1 : Switch  Criteria=u2 > Threshold  SaturateOnIntegerOverflow=off  InputSameDT=off
  SituationAwarness : Outport
  wires:
  In1/1 -> Bus Selector/1
  Constant/1 -> Switch/1
  Switch/1 -> Chart1/1(InScope)
  Constant1/1 -> Switch/3
  Bus Selector/1 -> Switch1/3, Switch/2  "<signal1>"
  Subsystem2/1(Aircraft#2Init) -> Bus Creator/2  "Aircraft#2Init"
  Bus Selector/2 -> Subsystem/1(In2)  "<signal2>"
  Subsystem/1(Aircraft#1Init) -> Bus Creator/1  "Aircraft#1Init"
  Subsystem3/1(Aircraft#3Init) -> Bus Creator/3  "Aircraft#3Init"
  Subsystem4/1(Aircraft#4Init) -> Bus Creator/4  "Aircraft#4Init"
  Subsystem5/1(Aircraft#5Init) -> Bus Creator/5  "Aircraft#5Init"
  Subsystem1/1(Aircraft#6Init) -> Bus Creator/6  "Aircraft#6Init"
  Chart1/1(Sensed) -> Switch1/2
  Bus Creator/1 -> SituationAwarness/1

== system AFASClosedloopSim/Servo ==
  ATServoCmd : Inport
  PitchServoCmd : Inport  Port=2
  RollServoCmd : Inport  Port=3
  YawServoCmd : Inport  Port=4
  Aileron: Actuation System Model : Subsystem
  Elevator: Actuation System Model : Subsystem
  Rudder: Actuation System Model : Subsystem
  Scope3 : Scope
  Throttle: Nonlinear Second-Order Actuator : aerolibactuator/Nonlinear Second-Order Actuator  wn_fin=1  z_fin=0.3  fin_max=20*pi/180  fin_min=-20*pi/180  fin_maxrate=500*pi/180  fin_act_0=0  fin_act_vel=0
  TLACmd : Outport
  ElevatorCmd : Outport  Port=2
  AileronCmd : Outport  Port=3
  RudderCmd : Outport  Port=4
  wires:
  ATServoCmd/1 -> Throttle: Nonlinear Second-Order Actuator/1
  Throttle: Nonlinear Second-Order Actuator/1 -> TLACmd/1
  PitchServoCmd/1 -> Elevator: Actuation System Model/1(motorPosCmd_rad)
  Elevator: Actuation System Model/1(elevPos_rad) -> ElevatorCmd/1
  RollServoCmd/1 -> Aileron: Actuation System Model/1(ailMotorPosCmd_rad)
  Aileron: Actuation System Model/1(tAilPos_rad) -> AileronCmd/1
  YawServoCmd/1 -> Rudder: Actuation System Model/1(rudMotorPosCmd_rad)
  Rudder: Actuation System Model/1(rudPos_rad) -> Scope3/1, RudderCmd/1

== system AFASClosedloopSim/UDP Sender ==
  OwnshipStates : Inport
  AIAircraft4DTCmd : Inport  Port=2
  Bus Selector : BusSelector  OutputSignals=Xe,Ye,Ze
  Byte Pack : etargetslib/Byte Pack  datatypes={'double','double','double','double','double'}  byteAlign=1
  Clock : Clock
  Out1 : Outport
  wires:
  OwnshipStates/1 -> Bus Selector/1
  Byte Pack/1 -> Out1/1
  Bus Selector/1 -> Byte Pack/1  "<Xe>"
  Bus Selector/2 -> Byte Pack/2  "<Ye>"
  Bus Selector/3 -> Byte Pack/3  "<Ze>"
  Clock/1 -> Byte Pack/4

== system AFASClosedloopSim/UDP receiver ==
  In1 : Inport
  Bus Creator : BusCreator  Inputs=3
  Bus Creator1 : BusCreator  Inputs=2
  Byte Unpack : etargetslib/Byte Unpack  dimensions={[1],[1],[1]}  datatypes={'double','double','double'}  byteAlign=1
      settings: LibrarySourceBlock=embeddedtargetslib/Host Communication/Byte Unpack
  Pi : Constant  Value=pi  OutDataTypeStr=Inherit: Inherit via back propagation
  Flight Rules : Outport
  AI aircraft Information : Outport  Port=2
  C2Link : Outport  Port=3
  wires:
  Byte Unpack/1 -> Bus Creator/2
  Byte Unpack/2 -> Bus Creator1/2
  Bus Creator/1 -> C2Link/1
  ? -> Flight Rules/1
  Pi/1 -> Bus Creator/1
  Byte Unpack/3 -> Bus Creator1/1
  Bus Creator1/1 -> AI aircraft Information/1

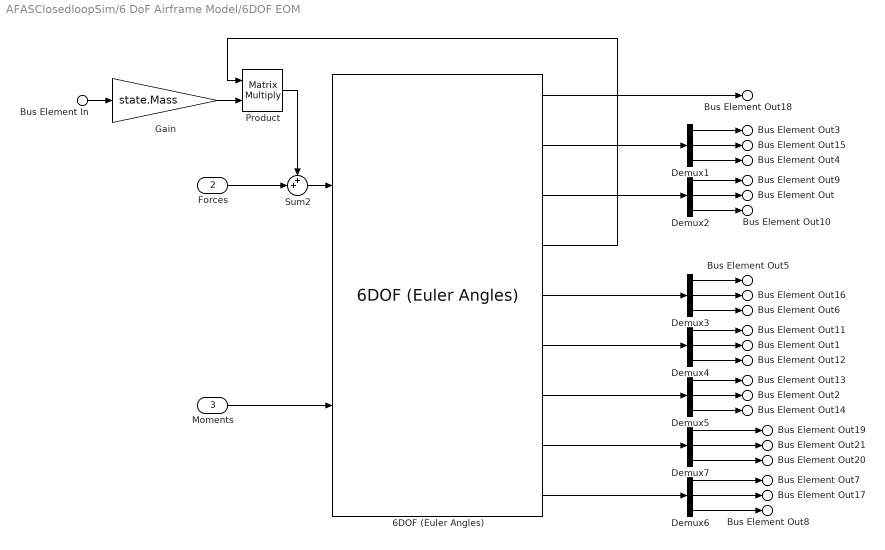
== system AFASClosedloopSim/6 DoF Airframe Model/6DOF EOM ==
  Bus Element In : Inport  PortName=Env  Element=g
  Forces : Inport  Port=2
  Moments : Inport  Port=3
  6DOF (Euler Angles) : shared6dof/6DOF (Euler Angles)  units=Metric (MKS)  mtype=Fixed  rep=Euler Angles  xme_0=[state.XN, state.XE, state.XD]  Vm_0=[state.U, state.V, state.W]  eul_0=[state.Phi, state.Theta, state.Psi]  pm_0=[state.P, state.Q, state.R]  mass_0=state.Mass  mass_e=0.5  mass_f=2.0  inertia=state.Inertia.Variables  inertia_e=eye(3)  inertia_f=2*eye(3)  k_quat=1.0  vre_flag=on  abi_flag=on  aMode=0  xme_statename={'Xe', 'Ye', 'Ze'}  Vm_statename={'U', 'V', 'W'}  eul_statename={'phi', 'theta', 'psi'}  quat_statename={'qr', 'qi', 'qj','qk'}  pm_statename={'p', 'q', 'r'}  mass_statename=''
  Demux{1..7} (7 alike) : Demux  Outputs=3
  Gain : Gain  Gain=state.Mass
  Product : Product  Multiplication=Matrix(*)
  Sum2 : Sum  Inputs=++|  InputSameDT=on  SaturateOnIntegerOverflow=on  OutDataTypeStr=Inherit: Same as first input
  Bus Element Out3 : Outport  VectorParamsAs1DForOutWhenUnconnected=off  PortName=States  Element=Xe
  Bus Element Out4 : Outport  VectorParamsAs1DForOutWhenUnconnected=off  PortName=States  Element=Ze
  Bus Element Out : Outport  VectorParamsAs1DForOutWhenUnconnected=off  PortName=States  Element=theta
  Bus Element Out5 : Outport  VectorParamsAs1DForOutWhenUnconnected=off  PortName=States  Element=u
  Bus Element Out6 : Outport  VectorParamsAs1DForOutWhenUnconnected=off  PortName=States  Element=w
  Bus Element Out1 : Outport  VectorParamsAs1DForOutWhenUnconnected=off  PortName=States  Element=q
  Bus Element Out2 : Outport  VectorParamsAs1DForOutWhenUnconnected=off  PortName=States  Element=q_dot
  Bus Element Out7 : Outport  VectorParamsAs1DForOutWhenUnconnected=off  PortName=States  Element=Axe
  Bus Element Out8 : Outport  VectorParamsAs1DForOutWhenUnconnected=off  PortName=States  Element=Aze
  Bus Element Out15 : Outport  VectorParamsAs1DForOutWhenUnconnected=off  PortName=States  Element=Ye
  Bus Element Out9 : Outport  VectorParamsAs1DForOutWhenUnconnected=off  PortName=States  Element=phi
  Bus Element Out10 : Outport  VectorParamsAs1DForOutWhenUnconnected=off  PortName=States  Element=psi
  Bus Element Out16 : Outport  VectorParamsAs1DForOutWhenUnconnected=off  PortName=States  Element=v
  Bus Element Out11 : Outport  VectorParamsAs1DForOutWhenUnconnected=off  PortName=States  Element=p
  Bus Element Out12 : Outport  VectorParamsAs1DForOutWhenUnconnected=off  PortName=States  Element=r
  Bus Element Out13 : Outport  VectorParamsAs1DForOutWhenUnconnected=off  PortName=States  Element=p_dot
  Bus Element Out14 : Outport  VectorParamsAs1DForOutWhenUnconnected=off  PortName=States  Element=r_dot
  Bus Element Out17 : Outport  VectorParamsAs1DForOutWhenUnconnected=off  PortName=States  Element=Aye
  Bus Element Out18 : Outport  VectorParamsAs1DForOutWhenUnconnected=off  PortName=States  Element=Ve
  Bus Element Out19 : Outport  VectorParamsAs1DForOutWhenUnconnected=off  PortName=States  Element=Axb
  Bus Element Out20 : Outport  VectorParamsAs1DForOutWhenUnconnected=off  PortName=States  Element=Azb
  Bus Element Out21 : Outport  VectorParamsAs1DForOutWhenUnconnected=off  PortName=States  Element=Ayb
  wires:
  6DOF (Euler Angles)/2 -> Demux1/1
  6DOF (Euler Angles)/4 -> Product/1
  6DOF (Euler Angles)/1 -> Bus Element Out18/1
  Bus Element In/1 -> Gain/1
  Demux6/2 -> Bus Element Out17/1
  Demux6/3 -> Bus Element Out8/1
  Demux6/1 -> Bus Element Out7/1
  6DOF (Euler Angles)/9 -> Demux6/1
  6DOF (Euler Angles)/7 -> Demux5/1
  Demux5/3 -> Bus Element Out14/1
  Demux5/2 -> Bus Element Out2/1
  Demux5/1 -> Bus Element Out13/1
  6DOF (Euler Angles)/6 -> Demux4/1
  Demux4/3 -> Bus Element Out12/1
  Demux4/2 -> Bus Element Out1/1
  Demux4/1 -> Bus Element Out11/1
  Demux3/3 -> Bus Element Out6/1
  Demux3/2 -> Bus Element Out16/1
  Demux3/1 -> Bus Element Out5/1
  6DOF (Euler Angles)/5 -> Demux3/1
  Demux2/3 -> Bus Element Out10/1
  Demux2/2 -> Bus Element Out/1
  Demux2/1 -> Bus Element Out9/1
  Demux1/1 -> Bus Element Out3/1
  Demux1/3 -> Bus Element Out4/1
  Demux1/2 -> Bus Element Out15/1
  Gain/1 -> Product/2
  6DOF (Euler Angles)/3 -> Demux2/1
  Moments/1 -> 6DOF (Euler Angles)/2
  Forces/1 -> Sum2/2
  Sum2/1 -> 6DOF (Euler Angles)/1
  Product/1 -> Sum2/1
  6DOF (Euler Angles)/8 -> Demux7/1
  Demux7/2 -> Bus Element Out21/1
  Demux7/1 -> Bus Element Out19/1
  Demux7/3 -> Bus Element Out20/1

== system AFASClosedloopSim/6 DoF Airframe Model/Aerodynamic Model ==
  Bus Element In13 : Inport  PortName=Env  Element=AirDensity
  Bus Element In14 : Inport  PortName=Env  Element=WindVelocity
  Bus Element In15 : Inport  PortName=Env  Element=WindAngularRates
  ActuatorCmds : Inport  Port=2
  Bus Element In1 : Inport  Port=3  PortName=States  Element=u
  Bus Element In2 : Inport  Port=3  PortName=States  Element=w
  Bus Element In3 : Inport  Port=3  PortName=States  Element=q
  Bus Element In6 : Inport  Port=3  PortName=States  Element=v
  Bus Element In4 : Inport  Port=3  PortName=States  Element=p
  Bus Element In5 : Inport  Port=3  PortName=States  Element=r
  Actuator Increments : Subsystem
  Aerodynamic Forces and Moments : aerolibadyn/Aerodynamic Forces and Moments   inputAxes=Body  outputForceAxes=Body  outputMomentAxes=Body  S=aircraft.ReferenceArea  b=aircraft.ReferenceSpan  cbar=aircraft.ReferenceLength
  Body Rate Damping : Subsystem
  Constant1 : Constant  Value=state.CenterOfGravity
  Constant2 : Constant  Value=state.CenterOfPressure
  Datum Coefficients : Subsystem
  Dynamic Pressure : aerolibasang/Dynamic Pressure
  Mux1 : Mux  Inputs=3
  Mux2 : Mux  Inputs=3
  Subsystem : Subsystem
  Sum1 : Sum  Inputs=-+|  InputSameDT=on  SaturateOnIntegerOverflow=on  OutDataTypeStr=Inherit: Same as first input
  Sum2 : Sum  Inputs=+++
  Sum3 : Sum  Inputs=|++  InputSameDT=on  SaturateOnIntegerOverflow=on  OutDataTypeStr=Inherit: Same as first input
  Terminator{,1..3} (4 alike) : Terminator
  ToBus : Subsystem
  F : Outport  Unit=N  VectorParamsAs1DForOutWhenUnconnected=off
  M : Outport  Port=2  Unit=N*m  VectorParamsAs1DForOutWhenUnconnected=off
  wires:
  Bus Element In14/1 -> Sum1/1
  Mux2/1 -> Sum1/2
  Mux1/1 -> Sum3/2
  Bus Element In15/1 -> Sum3/1
  Bus Element In5/1 -> Mux1/3
  Bus Element In3/1 -> Mux1/2
  Bus Element In4/1 -> Mux1/1
  Sum1/1 -> Dynamic Pressure/1, Subsystem/1(Vb)
  Dynamic Pressure/1 -> Aerodynamic Forces and Moments/2  "qbar"
  Sum3/1 -> ToBus/1(I)
  Bus Element In13/1 -> Dynamic Pressure/2
  Aerodynamic Forces and Moments/2 -> M/1
  Aerodynamic Forces and Moments/1 -> F/1
  Constant2/1 -> Aerodynamic Forces and Moments/4
  Constant1/1 -> Aerodynamic Forces and Moments/3
  Sum2/1 -> Aerodynamic Forces and Moments/1
  Bus Element In1/1 -> Mux2/1
  Bus Element In6/1 -> Mux2/2
  Bus Element In2/1 -> Mux2/3
  Subsystem/1(Alpha) -> Datum Coefficients/1(alpha), Actuator Increments/1(alpha)
  Subsystem/4(Beta) -> Datum Coefficients/2(beta), Actuator Increments/2(beta)
  Actuator Increments/1(Coefficients) -> Sum2/1
  ActuatorCmds/1 -> Actuator Increments/3(ActuatorCmds)
  Datum Coefficients/1(Coefficients) -> Sum2/2
  Body Rate Damping/1(Coefficients) -> Sum2/3
  ToBus/1(O) -> Body Rate Damping/2(p,q,r)
  Subsystem/7(V) -> Body Rate Damping/1(V)
  Subsystem/2(Alpha2) -> Terminator/1
  Subsystem/6(Beta3) -> Terminator3/1
  Subsystem/5(Beta2) -> Terminator1/1
  Subsystem/3(Alpha3) -> Terminator2/1

== system AFASClosedloopSim/6 DoF Airframe Model/Environment Model ==
  Bus Element In1 : Inport  PortName=States  Element=u
  Bus Element In2 : Inport  PortName=States  Element=w
  Bus Element In3 : Inport  PortName=States  Element=theta
  Bus Element In4 : Inport  PortName=States  Element=Xe
  Bus Element In7 : Inport  PortName=States  Element=Ze
  Bus Element In8 : Inport  PortName=States  Element=phi
  Bus Element In5 : Inport  PortName=States  Element=psi
  Bus Element In6 : Inport  PortName=States  Element=Ye
  COESA Atmosphere Model : aerolibatmos2/COESA Atmosphere Model  units=Metric (MKS)  spec=1976 COESA-extended U.S. Standard Atmosphere  model=Profile  profile_var=High temperature  profile_percent=1%  profile_alt=5 km (16404 ft)  envelope_var=High temperature  envelope_percent=1%  action=Warning
  Dryden Wind Turbulence Model (Continuous (+q +r)) : aerolibwind2/Dryden Wind Turbulence Model  (Continuous (+q -r))  units=Metric (MKS)  spec=MIL-F-8785C  model=Continuous Dryden (+q -r)  W20=W20  Wdeg=Wdeg  TurbProb=10^-2 - Light  L_high=L_high  Wingspan=Wingspan  ts=ts  Seed=Seed  T_on=off
  Earth Reference Alt : Constant  Value=refAlt
  Flat Earth to LLA : aerolibtransform2/Flat Earth to LLA  units=Metric (MKS)  ptype=Earth (WGS84)  F=1/298.257223563  R=6378137  refPosPort=off  LL0=[0 0]  psi=0
  Incidence & Airspeed : aerolibasang/Incidence  & Airspeed
  Mux : Mux  Inputs=3
  Mux1 : Mux  Inputs=3
  Mux2 : Mux  Inputs=2
  Mux3 : Mux  Inputs=2
  Rotation Angles to Direction Cosine Matrix : sharedtransform/Rotation Angles to Direction Cosine Matrix  rotationOrder=ZYX  aMode=aMode
  Terminator : Terminator
  "WGS84 Gravity Model  " : GravityWGS84
  Bus Element Out : Outport  VectorParamsAs1DForOutWhenUnconnected=off  PortName=Env  Element=To
  Bus Element Out1 : Outport  VectorParamsAs1DForOutWhenUnconnected=off  PortName=Env  Element=a
  Bus Element Out2 : Outport  VectorParamsAs1DForOutWhenUnconnected=off  PortName=Env  Element=Po
  Bus Element Out3 : Outport  VectorParamsAs1DForOutWhenUnconnected=off  PortName=Env  Element=AirDensity
  Bus Element Out4 : Outport  VectorParamsAs1DForOutWhenUnconnected=off  PortName=Env  Element=WindVelocity
  Bus Element Out5 : Outport  VectorParamsAs1DForOutWhenUnconnected=off  PortName=Env  Element=WindAngularRates
  Bus Element Out6 : Outport  VectorParamsAs1DForOutWhenUnconnected=off  PortName=Env  Element=g
  wires:
  Dryden Wind Turbulence Model (Continuous (+q +r))/1 -> Bus Element Out4/1
  Dryden Wind Turbulence Model (Continuous (+q +r))/2 -> Bus Element Out5/1
  Mux2/1 -> "WGS84 Gravity Model  "/1
  Bus Element In4/1 -> Mux1/1
  Bus Element In7/1 -> Mux1/3
  Bus Element In6/1 -> Mux1/2
  Bus Element In5/1 -> Mux/3
  Bus Element In8/1 -> Mux/1
  Bus Element In2/1 -> Mux3/2
  Bus Element In1/1 -> Mux3/1
  "WGS84 Gravity Model  "/1 -> Bus Element Out6/1
  COESA Atmosphere Model/2 -> Bus Element Out1/1
  COESA Atmosphere Model/1 -> Bus Element Out/1
  COESA Atmosphere Model/4 -> Bus Element Out3/1
  COESA Atmosphere Model/3 -> Bus Element Out2/1
  Flat Earth to LLA/1 -> Mux2/1
  Earth Reference Alt/1 -> Flat Earth to LLA/2
  Incidence & Airspeed/2 -> Dryden Wind Turbulence Model (Continuous (+q +r))/2
  Flat Earth to LLA/2 -> Mux2/2, COESA Atmosphere Model/1, Dryden Wind Turbulence Model (Continuous (+q +r))/1
  Mux3/1 -> Incidence & Airspeed/1
  Incidence & Airspeed/1 -> Terminator/1
  Mux/1 -> Rotation Angles to Direction Cosine Matrix/1
  Bus Element In3/1 -> Mux/2
  Rotation Angles to Direction Cosine Matrix/1 -> Dryden Wind Turbulence Model (Continuous (+q +r))/3
  Mux1/1 -> Flat Earth to LLA/1

== system AFASClosedloopSim/6 DoF Airframe Model/Propulsion ==
  cmd : Inport
  Mux : Mux  Inputs=[1 2]
  ThrustYZ : Constant  Value=[0 0]'  SampleTime=-1
  Thrust_M1 : Constant  Value=[0 0 0]'  SampleTime=-1
  F : Outport  Unit=N  VectorParamsAs1DForOutWhenUnconnected=off
  M : Outport  Port=2  Unit=N*m  VectorParamsAs1DForOutWhenUnconnected=off
  wires:
  Thrust_M1/1 -> M/1
  cmd/1 -> Mux/1
  ThrustYZ/1 -> Mux/2
  Mux/1 -> F/1

== system AFASClosedloopSim/6 DoF Airframe Model/Visualization ==
  Bus Element In : Inport  PortName=States  Element=u
  Bus Element In1 : Inport  PortName=States  Element=w
  Bus Element In3 : Inport  PortName=States  Element=q
  Bus Element In4 : Inport  PortName=States  Element=theta
  Bus Element In12 : Inport  PortName=States  Element=Ze
  Bus Element In2 : Inport  PortName=States  Element=Xe
  Bus Element In10 : Inport  PortName=States  Element=v
  Bus Element In5 : Inport  PortName=States  Element=phi
  Bus Element In6 : Inport  PortName=States  Element=psi
  Bus Element In7 : Inport  PortName=States  Element=p
  Bus Element In8 : Inport  PortName=States  Element=r
  Bus Element In9 : Inport  PortName=States  Element=Ye
  "Incidence, Sideslip, & Airspeed" : aerolibasang/Incidence, Sideslip, & Airspeed
  Mux{1..4} (4 alike) : Mux  Inputs=3
  Mux5 : Mux  Inputs=2
  State Plots : Scope  NumInputPorts=4
  Terminator : Terminator
  wires:
  Mux3/1 -> State Plots/4
  Bus Element In2/1 -> Mux3/1  "Xe"
  Bus Element In9/1 -> Mux3/2  "Ye"
  Bus Element In12/1 -> Mux3/3  "Ze"
  Mux2/1 -> State Plots/3
  Mux1/1 -> State Plots/2
  Mux5/1 -> State Plots/1
  "Incidence, Sideslip, & Airspeed"/2 -> Mux5/2  "beta"
  "Incidence, Sideslip, & Airspeed"/1 -> Mux5/1  "alpha"
  Mux4/1 -> "Incidence, Sideslip, & Airspeed"/1
  Bus Element In10/1 -> Mux4/2
  Bus Element In8/1 -> Mux2/3  "r"
  Bus Element In7/1 -> Mux2/1  "p"
  Bus Element In6/1 -> Mux1/3  "psi"
  Bus Element In5/1 -> Mux1/1  "phi"
  Bus Element In4/1 -> Mux1/2  "theta"
  Bus Element In3/1 -> Mux2/2  "q"
  Bus Element In1/1 -> Mux4/3
  Bus Element In/1 -> Mux4/1
  "Incidence, Sideslip, & Airspeed"/3 -> Terminator/1

== system AFASClosedloopSim/AFAS has four sub-moduels: 1) Detect and Avoid (DAA); 2) Aircraft Separation Assurance System (ASAS); 3) Collaborative Decision Assistance System (CDAS); 4) Decentralized Decision Assistance System (DDAS) /ASAS: Aircraft Separation Assurance System ==
  In1 : Inport
  Out1 : Outport
  wires:
  In1/1 -> Out1/1

== system AFASClosedloopSim/AFAS has four sub-moduels: 1) Detect and Avoid (DAA); 2) Aircraft Separation Assurance System (ASAS); 3) Collaborative Decision Assistance System (CDAS); 4) Decentralized Decision Assistance System (DDAS) /CDAS: Collaborative Decision Assistance System ==
  In1 : Inport
  Out1 : Outport
  wires:
  In1/1 -> Out1/1

== system AFASClosedloopSim/AFAS has four sub-moduels: 1) Detect and Avoid (DAA); 2) Aircraft Separation Assurance System (ASAS); 3) Collaborative Decision Assistance System (CDAS); 4) Decentralized Decision Assistance System (DDAS) /DAA: Detection and Avoid ==
  In1 : Inport
  Out1 : Outport
  wires:
  In1/1 -> Out1/1

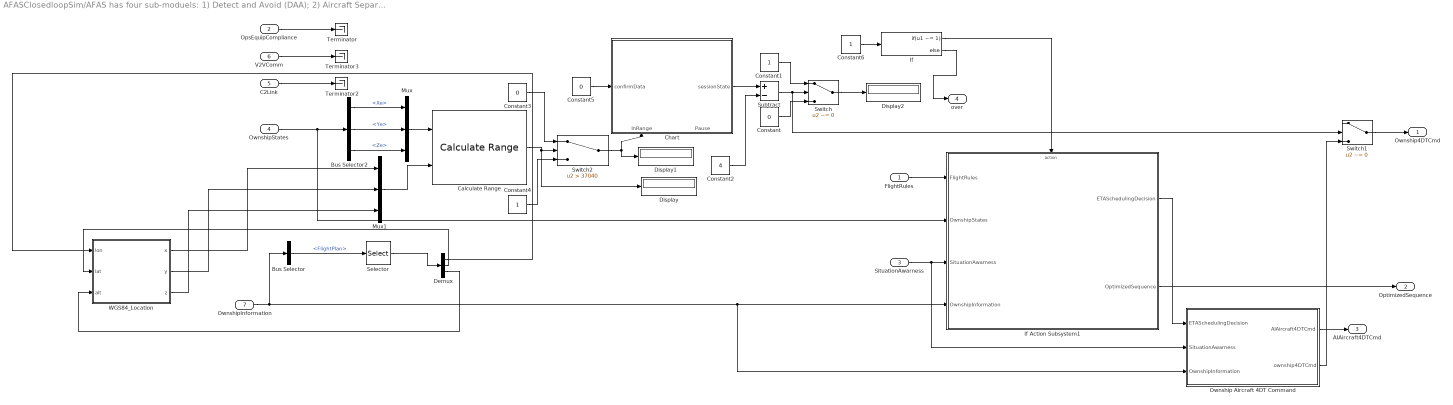
== system AFASClosedloopSim/AFAS has four sub-moduels: 1) Detect and Avoid (DAA); 2) Aircraft Separation Assurance System (ASAS); 3) Collaborative Decision Assistance System (CDAS); 4) Decentralized Decision Assistance System (DDAS) /DDAS: Decentralized Decision Assistance System ==
  FlightRules : Inport
  OpsEquipCompliance : Inport  Port=2
  SituationAwarness : Inport  Port=3
  OwnshipStates : Inport  Port=4
  C2Link : Inport  Port=5
  V2VComm : Inport  Port=6
  OwnshipInformation : Inport  Port=7
  Bus Selector : BusSelector  OutputSignals=FlightPlan
  Bus Selector2 : BusSelector  OutputSignals=Xe,Ye,Ze
  Calculate Range : aerolibguid/Calculate Range
  Chart : Stateflow chart  TreatAsAtomicUnit=on
      settings: PortSchema="{\"entries\":[{\"content\":{\"sides\":[{\"content\":{\"connectorIds\":[\"In1\"]},\"type\":\"ConnectorPlacement.EquallySpacedRectSide\",\"uuid\":\"0168b176-f8da-4a18-91c2-56ac9a2470ea\"},{\"content\":{\"connectorIds\":[\"Out1\"],\"side\":\"RIGHT\"},\"type\":\"ConnectorPlacement.EquallySpacedRectSide\",\"uuid\":\"ec5b6235-baf8-4595-b51b-352b99491068\"},{\"content\":{\"side\":\"TOP\"},\"type\":\"ConnectorPlacement.EquallySpacedRectSide\",\"uuid\":\"fe57ce38-d401-441f-9cd7-d99e4b878af8\"},{\"content\":{\"connectorIds\":[\"In2\",\"In3\"],\"side\":\"BOTTOM\"},\"type\":\"ConnectorPlacement.EquallySpacedRectSide\",\"uuid\":\"923392b6-0697-43e9-840b-49860b5d5671\"}]},\"type\":\"ConnectorPlacement.EquallySpacedConnector\",\"uuid\":\"e4cb718f-1761-4aa5-94ee-8fd0b5f5d55e\"}],\"packageUris\":[\"http://schema.mathworks.com/mf0/Connector/R2020b\"],\"version\":\"1.0\"}"
  Constant : Constant  Value=0
  Constant1 : Constant
  Constant2 : Constant  Value=4
  Constant3 : Constant  Value=0
  Constant4 : Constant
  Constant5 : Constant  Value=0
  Constant6 : Constant
  Demux : Demux  Outputs=3
  Display : Display
  Display1 : Display
  Display2 : Display
  If : If  IfExpression=u1 ~= 1
  If Action Subsystem1 : Subsystem  TreatAsAtomicUnit=on
  Mux : Mux  Inputs=3
  Mux1 : Mux  Inputs=3
  Ownship Aircraft 4DT Command : Subsystem
  Selector : Selector  NumberOfDimensions=2  InputPortWidth=4  IndexOptions=Index vector (dialog),Index vector (dialog)  Indices=[1],[1,2,3]  OutputSizes=1,1
  Subtract : Sum  Inputs=+-
  Switch : Switch  Criteria=u2 ~= 0  SaturateOnIntegerOverflow=off  InputSameDT=off
  Switch1 : Switch  Criteria=u2 ~= 0  SaturateOnIntegerOverflow=off  InputSameDT=off
  Switch2 : Switch  Criteria=u2 > Threshold  Threshold=37040  SaturateOnIntegerOverflow=off  InputSameDT=off
  Terminator : Terminator
  Terminator2 : Terminator
  Terminator3 : Terminator
  WGS84_Location : Subsystem
  Ownship4DTCmd : Outport
  OptimizedSequence : Outport  Port=2
  AIAircraft4DTCmd : Outport  Port=3
  over : Outport  Port=4
  wires:
  V2VComm/1 -> Terminator3/1
  OpsEquipCompliance/1 -> Terminator/1
  Calculate Range/1 -> Display/1, Switch2/2
  C2Link/1 -> Terminator2/1
  OwnshipStates/1 -> Bus Selector2/1, If Action Subsystem1/2(OwnshipStates)
  Bus Selector2/1 -> Mux/1  "<Xe>"
  OwnshipInformation/1 -> Bus Selector/1, Ownship Aircraft 4DT Command/3(OwnshipInformation), If Action Subsystem1/4(OwnshipInformation)
  Constant3/1 -> Switch2/1
  Constant4/1 -> Switch2/3
  If/1 -> If Action Subsystem1/Action
  Switch2/1 -> Display1/1, Chart/2(InRange)
  Chart/1(sessionState) -> Subtract/1
  Constant2/1 -> Subtract/2
  Constant1/1 -> Switch/1
  Subtract/1 -> Switch1/2, Switch/2
  If Action Subsystem1/2(OptimizedSequence) -> OptimizedSequence/1
  Constant/1 -> Switch/3
  If/2 -> over/1
  FlightRules/1 -> If Action Subsystem1/1(FlightRules)
  SituationAwarness/1 -> Ownship Aircraft 4DT Command/2(SituationAwarness), If Action Subsystem1/3(SituationAwarness)
  If Action Subsystem1/1(ETASchedulingDecision) -> Ownship Aircraft 4DT Command/1(ETASchedulingDecision)
  Ownship Aircraft 4DT Command/1(AIAircraft4DTCmd) -> AIAircraft4DTCmd/1
  Ownship Aircraft 4DT Command/2(ownship4DTCmd) -> Switch1/3
  Switch1/1 -> Ownship4DTCmd/1
  Bus Selector2/2 -> Mux/2  "<Ye>"
  Bus Selector2/3 -> Mux/3  "<Ze>"
  Mux/1 -> Calculate Range/1
  Bus Selector/1 -> Selector/1  "<FlightPlan>"
  Demux/2 -> WGS84_Location/2(lat)
  Selector/1 -> Demux/1
  Demux/1 -> WGS84_Location/1(lon)
  Demux/3 -> WGS84_Location/3(alt)
  Mux1/1 -> Calculate Range/2
  WGS84_Location/1(x) -> Mux1/1
  WGS84_Location/2(y) -> Mux1/2
  WGS84_Location/3(z) -> Mux1/3
  Constant5/1 -> Chart/1(confirmData)
  Switch/1 -> Display2/1
  Constant6/1 -> If/1
